simulink model "Function_Blocks"  (R2020b)
settings: Solver=FixedStepDiscrete  StartTime=0.0  StopTime=40  FixedStep=0.001  RelTol=1e-3
undefined symbols (not defined in the file): AA, C1, DiscIntNeverNeededParam, Error_Limit, kq, kqL
libraries: simulink x1, eeGeneralControl x1
(part 2 of 2)

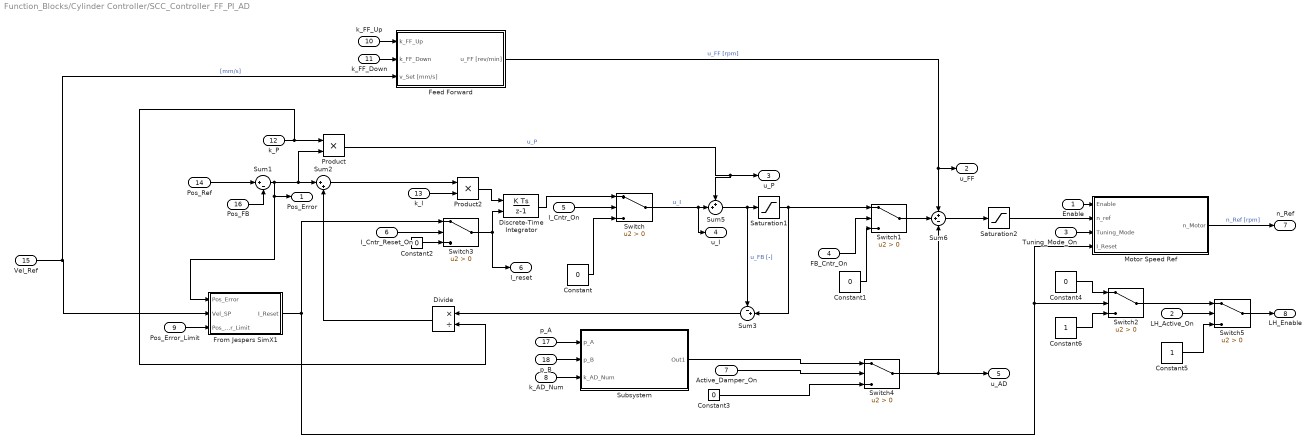
== system Function_Blocks/Cylinder Controller/SCC_Controller_FF_PI_AD ==
  Enable : Inport  OutDataTypeStr=boolean
  LH_Active_On : Inport  Port=2
  Tuning_Mode_On : Inport  Port=3  OutDataTypeStr=boolean
  FB_Cntr_On : Inport  Port=4  OutDataTypeStr=boolean
  I_Cntr_On : Inport  Port=5  OutDataTypeStr=boolean
  I_Cntr_Reset_On : Inport  Port=6  OutDataTypeStr=boolean
  Active_Damper_On : Inport  Port=7  OutDataTypeStr=boolean
  k_AD_Num : Inport  Port=8
  Pos_Error_Limit : Inport  Port=9
  k_FF_Up : Inport  Port=10
  k_FF_Down : Inport  Port=11
  k_P : Inport  Port=12
  k_I : Inport  Port=13
  Pos_Ref : Inport  Port=14
  Vel_Ref : Inport  Port=15
  Pos_FB : Inport  Port=16
  p_A : Inport  Port=17
  p_B : Inport  Port=18
  Constant{,1..3} (4 alike) : Constant  Value=0
  Constant4 : Constant  Value=0  OutDataTypeStr=boolean
  Constant5 : Constant  OutDataTypeStr=boolean
  Constant6 : Constant  OutDataTypeStr=boolean
  Discrete-Time Integrator : DiscreteIntegrator  ExternalReset=sampled level  SampleTime=0.001  ICPrevOutput=DiscIntNeverNeededParam  ICPrevScaledInput=DiscIntNeverNeededParam
  Divide : Product  Inputs=*/
  Feed Forward : Subsystem
  From Jespers SimX1 : MATLAB Function  TreatAsAtomicUnit=on
  Motor Speed Ref : MATLAB Function  TreatAsAtomicUnit=on
  Product : Product
  Product2 : Product
  Saturation1 : Saturate  UpperLimit=3500  LowerLimit=-3500
  Saturation2 : Saturate  UpperLimit=3500  LowerLimit=-3500
  Subsystem : Subsystem
  Sum1 : Sum  Inputs=|+-
  Sum2 : Sum  Inputs=|++
  Sum3 : Sum  Inputs=-+|
  Sum5 : Sum  Inputs=++|
  Sum6 : Sum  Inputs=++-
  Switch{,1..5} (6 alike) : Switch  Criteria=u2 > Threshold
  Pos_Error : Outport  VectorParamsAs1DForOutWhenUnconnected=off
  u_FF : Outport  Port=2  VectorParamsAs1DForOutWhenUnconnected=off
  u_P : Outport  Port=3  VectorParamsAs1DForOutWhenUnconnected=off
  u_I : Outport  Port=4  VectorParamsAs1DForOutWhenUnconnected=off
  u_AD : Outport  Port=5  VectorParamsAs1DForOutWhenUnconnected=off
  I_reset : Outport  Port=6  VectorParamsAs1DForOutWhenUnconnected=off
  n_Ref : Outport  Port=7  VectorParamsAs1DForOutWhenUnconnected=off
  LH_Enable : Outport  Port=8  OutDataTypeStr=boolean  VectorParamsAs1DForOutWhenUnconnected=off
  wires:
  Product2/1 -> Discrete-Time Integrator/1
  Pos_FB/1 -> Sum1/2
  Product/1 -> u_P/1, Sum5/1  "u_P"
  Sum2/1 -> Product2/1
  Divide/1 -> Sum2/2
  k_P/1 -> Divide/2, Product/1
  k_I/1 -> Product2/2
  Sum1/1 -> From Jespers SimX1/1(Pos_Error), Pos_Error/1, Product/2, Sum2/1
  Discrete-Time Integrator/1 -> Switch/1
  Switch/1 -> u_I/1, Sum5/2  "u_I"
  I_Cntr_On/1 -> Switch/2
  Constant/1 -> Switch/3
  Pos_Ref/1 -> Sum1/1
  Vel_Ref/1 -> Feed Forward/3(v_Set [mm/s]), From Jespers SimX1/2(Vel_SP)  "[mm/s]"
  Switch3/1 -> I_reset/1, Discrete-Time Integrator/2
  Saturation2/1 -> Motor Speed Ref/2(n_ref)
  Sum5/1 -> Sum3/1, Saturation1/1  "u_FB [-]"
  I_Cntr_Reset_On/1 -> Switch3/2
  Pos_Error_Limit/1 -> From Jespers SimX1/3(Pos_Error_Limit)
  Constant2/1 -> Switch3/3
  Constant3/1 -> Switch4/3
  Active_Damper_On/1 -> Switch4/2
  Switch4/1 -> Sum6/3, u_AD/1
  p_A/1 -> Subsystem/1(p_A)
  p_B/1 -> Subsystem/2(p_B)
  k_AD_Num/1 -> Subsystem/3(k_AD_Num)
  Subsystem/1(Out1) -> Switch4/1
  Tuning_Mode_On/1 -> Motor Speed Ref/3(Tuning_Mode)
  Motor Speed Ref/1(n_Motor) -> n_Ref/1  "n_Ref [rpm]"
  Sum3/1 -> Divide/1
  Sum6/1 -> Saturation2/1
  Feed Forward/1(u_FF [rev/min]) -> u_FF/1, Sum6/1  "u_FF [rpm]"
  Constant1/1 -> Switch1/3
  FB_Cntr_On/1 -> Switch1/2
  Saturation1/1 -> Switch1/1, Sum3/2
  Switch1/1 -> Sum6/2
  Constant5/1 -> Switch5/3
  LH_Active_On/1 -> Switch5/2
  Switch5/1 -> LH_Enable/1
  Enable/1 -> Motor Speed Ref/1(Enable)
  k_FF_Up/1 -> Feed Forward/1(k_FF_Up)
  k_FF_Down/1 -> Feed Forward/2(k_FF_Down)
  From Jespers SimX1/1(I_Reset) -> Switch2/2, Motor Speed Ref/4(I_Reset), Switch3/1
  Switch2/1 -> Switch5/1
  Constant4/1 -> Switch2/1
  Constant6/1 -> Switch2/3

== system Function_Blocks/Pressure_Feed_Forward/Subsystem2 ==
  p001 : Inport
  Trigger : TriggerPort  TriggerType=falling  VariantControl=Variant  PortDimensions=1
  p001_Hold : Outport  VectorParamsAs1DForOutWhenUnconnected=off
  wires:
  p001/1 -> p001_Hold/1

== system Function_Blocks/SCC_DPF/Subsystem ==
  pp : Inport
  pr : Inport  Port=2
  Trigger : TriggerPort  TriggerType=falling  VariantControl=Variant  PortDimensions=1
  pp0 : Outport  VectorParamsAs1DForOutWhenUnconnected=off
  pr0 : Outport  Port=2  VectorParamsAs1DForOutWhenUnconnected=off
  wires:
  pp/1 -> pp0/1
  pr/1 -> pr0/1

== system Function_Blocks/SCC_HPPF1/Subsystem2 ==
  pp : Inport
  pr : Inport  Port=2
  Trigger : TriggerPort  TriggerType=falling  VariantControl=Variant  PortDimensions=1
  pp0 : Outport  VectorParamsAs1DForOutWhenUnconnected=off
  pr0 : Outport  Port=2  VectorParamsAs1DForOutWhenUnconnected=off
  wires:
  pp/1 -> pp0/1
  pr/1 -> pr0/1

== system Function_Blocks/SCC_LPPF/Subsystem ==
  pp : Inport
  pr : Inport  Port=2
  Trigger : TriggerPort  TriggerType=falling  VariantControl=Variant  PortDimensions=1
  pp0 : Outport  VectorParamsAs1DForOutWhenUnconnected=off
  pr0 : Outport  Port=2  VectorParamsAs1DForOutWhenUnconnected=off
  wires:
  pp/1 -> pp0/1
  pr/1 -> pr0/1

== system Function_Blocks/Cylinder Controller/SCC_Controller_FF_PI_AD/Feed Forward ==
  k_FF_Up : Inport
  k_FF_Down : Inport  Port=2
  v_Set [mm/s] : Inport  Port=3
  Lift crane (pumping mode) : Product
  Lower crane (motoring mode) : Product
  Switch : Switch
  u_FF [rev/min] : Outport  VectorParamsAs1DForOutWhenUnconnected=off
  wires:
  Lower crane (motoring mode)/1 -> Switch/3  "[rev/min]"
  Lift crane (pumping mode)/1 -> Switch/1  "[rev/min]"
  Switch/1 -> u_FF [rev/min]/1
  v_Set [mm/s]/1 -> Lower crane (motoring mode)/1, Lift crane (pumping mode)/2, Switch/2
  k_FF_Up/1 -> Lift crane (pumping mode)/1
  k_FF_Down/1 -> Lower crane (motoring mode)/2

== system Function_Blocks/Cylinder Controller/SCC_Controller_FF_PI_AD/Subsystem ==
  p_A : Inport
  p_B : Inport  Port=2
  k_AD_Num : Inport  Port=3
  Cylinder Area Ratio : Gain  Gain=0.710059171597633
  Gain1 : Gain  Gain=-1
  Load Pressure : Sum  Inputs=|+-  OutDataTypeStr=double
  Scope : Scope
  Transfer Fcn1 1 : DiscreteTransferFcn  NumeratorSource=Input port  Numerator=[5e-5 -5e-05]  Denominator=[1 -0.997]  a0EqualsOne=on
      settings: InputPortMap=u0,p1
  Vector Concatenate : Concatenate
  Out1 : Outport  VectorParamsAs1DForOutWhenUnconnected=off
  wires:
  k_AD_Num/1 -> Vector Concatenate/1, Gain1/1
  Transfer Fcn1 1/1 -> Out1/1, Scope/1
  p_A/1 -> Load Pressure/1
  Vector Concatenate/1 -> Transfer Fcn1 1/2
  Cylinder Area Ratio/1 -> Load Pressure/2
  Load Pressure/1 -> Transfer Fcn1 1/1
  p_B/1 -> Cylinder Area Ratio/1
  Gain1/1 -> Vector Concatenate/2

== matlab function Function_Blocks/SCC_SinProfile/WaveSignal ==
  data: x0 input; v0 input; xC_SP input; Ts input; phi input; x output; t input; dx output
function [x,dx] = fcn(x0,v0,xC_SP,Ts,phi,t)

A=xC_SP/2;

x0=x0+A;
v0=v0;

x = x0+A*cos(2*pi*(1/Ts)*t+phi);
dx = v0-2*pi*A*(1/Ts)*sin(2*pi*(1/Ts)*t+phi);

== matlab function Function_Blocks/SCC_Cascaded_Controller/Controller_Reset ==
  data: Clock input; I_Reset output
function I_Reset = fcn(Clock)

I_Reset = 1;

if Clock > 0
   I_Reset = 0;
else
    I_Reset = 1;
end

== matlab function Function_Blocks/LHV_Enabler/MATLAB Function1 ==
  data: y output; LHC_error input; LHC_error_SP input; SM_ON input
function y = fcn(LHC_error, LHC_error_SP, SM_ON)


if SM_ON > 0 && abs(LHC_error)  < LHC_error_SP
y = 1;  
else 
y = 0;
end

== matlab function Function_Blocks/Pressure_Feed_Forward/MATLAB Function1 ==
  data: FeedBackPressureTerm output; p001_Hold input; p_32 input; x_dot_ref input
function FeedBackPressureTerm = fcn(p001_Hold,p_32,x_dot_ref)

if (p001_Hold - p_32) <= 0
FeedBackPressureTerm = 0;
elseif abs(x_dot_ref) > 0.0003
FeedBackPressureTerm = 0;
else
FeedBackPressureTerm =  6.0256*10^(-5)/2 * (p001_Hold - p_32);
end

== matlab function Function_Blocks/VCC_Pos_Step/StepFunction ==
  data: x0 input; x_SP input; t0 input; t1 input; t input; y output
function y  = step(x0,x_SP, t0,t1,  t)


if t>=0 && t<t0
    y = x0;
elseif t>=(t0) && t<(t0+t1)
    y = x_SP;
else
    y = x0; 
end

== matlab function Function_Blocks/S_shape_Profile/SP_Generator ==
  data: PositionRef output; VelocityRef output; AccelerationRef output; JerkRef output; InPositionTime output; s0 input; v0 input; Desired_Position input; VelocitySP input; t0 input; HoldPositionTime input; t input; Error output
function [PositionRef,VelocityRef,AccelerationRef,JerkRef, InPositionTime, Error] = fcn(s0,v0, Desired_Position,VelocitySP, t0,HoldPositionTime,t)


PositionSP = Desired_Position - s0;

a0 = 0;
j0 = 0;
AccelerationSP = VelocitySP;

vel=VelocitySP;
as=AccelerationSP;
% Input velocity 
vs=vel; %[rad/s]
% Delta velocity 
dv=(vs-v0); %[rad/s]     
% Max Jerk Considerations
jm=as^2/dv; %%[rad/s^3] 
% Constant Velocity periodes
s_acc=(vs^2-v0^2)/as;
CstVelTime=(PositionSP-2*s_acc)/vs;
if CstVelTime < 0
Error = 1;
else 
Error = 0;
end

% Time periodes,
t1=t0+(as/jm);
t2=t1+(as/jm);
t3=t2+CstVelTime;
t4=t3+(as/jm);
t5=t4+(as/jm);
t6=t5+HoldPositionTime;
t7=t6+(as/jm);
t8=t7+(as/jm);
t9=t8+CstVelTime;
t10=t9+(as/jm);
t11=t10+(as/jm);
% Position and Velocity Constants
sh=(v0+(as^2)/(6*jm))*(as/jm);
vh=(vs-v0)/2;
s3=s_acc+vs*(t3-t2);
s4=s3+vs*(t4-t3)-jm*((t4-t3)^3)/6;
v4=vs-jm*((t4-t3)^2)/2;
s5=s0+jm*((t5-t4)^3)/6-as*((t5-t4)^2)/2+v4*(t5-t4)+s4;
%s6=s5+(s0+v0*(t7-t6)+jm*((t7-t6)^3)/6);
s7= s5-(s_acc+vs*(t9-t8));
s8= s7-(vs*(t10-t9)-jm*((t10-t9)^3)/6);
%s9= s8-(jm*((t11-t10)^3)/6-as*((t11-t10)^2)/2+v4*(t11-t10));
%Phase0
if  Error == 1   
s = s0;
v = v0;
a = a0;
j=j0; 
elseif  (t >= 0) && (t <= t0)    
s = s0;
v = v0;
a = a0;
j=j0;        
%Phase1 - concave Acc
elseif  (t >= t0) && (t <= (t1))
s = s0+v0*(t-t0)+jm*((t-t0)^3)/6;
v = v0+jm*((t-t0)^2)/2;
a = jm*(t-t0);
j=jm;
%Phase2 - convex Acc
elseif (t >= (t1)) && (t <= (t2))
s = s0+sh+vh*(t-t1)+as*((t-t1)^2)/2-jm*((t-t1)^3)/6;
v = vh+as*(t-t1)-jm*((t-t1)^2)/2;
a = as-jm*(t-t1);
j = -jm; 
%Phase3 - constant velocity
elseif (t >= t2) && (t <= t3)
s = s0+s_acc+vs*(t-t2);
v = vs;
a = 0;
j = 0;   
%Phase4 - convex Dec
elseif (t >= t3) && (t <= t4)
s = s0+s3+vs*(t-t3)-jm*((t-t3)^3)/6;
v = vs-jm*((t-t3)^2)/2;
a = -jm*(t-t3);
j = -jm; 
%Phase5 - concav Dec
elseif (t >= t4) && (t <= t5)
s = s0+jm*((t-t4)^3)/6-as*((t-t4)^2)/2+v4*(t-t4)+s4;
v = jm*((t-t4)^2)/2-as*(t-t4)+v4;
a = jm*(t-t4)-as;
j=jm; 
%Phase6 - holding position
elseif (t >= t5) && (t <= t6)
s = s5;
v = 0;
a = 0;
j = 0;  
%Phase7 - concave Dec
elseif (t >= t6) && (t <= t7)
s = s5-(v0*(t-t6)+jm*((t-t6)^3)/6);
v = -(v0+jm*((t-t6)^2)/2);
a = -jm*(t-t6);
j=-jm;
%Phase8 - convex Dec
elseif (t >= t7) && (t <= t8)    
s = s5-(sh+vh*(t-t7)+as*((t-t7)^2)/2-jm*((t-t7)^3)/6);
v = -(vh+as*(t-t7)-jm*((t-t7)^2)/2);
a = -(as-jm*(t-t7));
j = jm; 
%Phase9 - constant velocity
elseif (t >= t8) && (t <= t9)
s = s5-(s_acc+vs*(t-t8));
v = -vs;
a = 0;
j = 0;     
%Phase10 - concav Acc
elseif (t >= t9) && (t <= t10)
s = s7-(vs*(t-t9)-jm*((t-t9)^3)/6);
v = -(vs-jm*((t-t9)^2)/2);
a = jm*(t-t9);
j = jm; 
%Phase11 - convex Acc
elseif (t >= t10) && (t <= t11)
s = s8-(jm*((t-t10)^3)/6-as*((t-t10)^2)/2+v4*(t-t10));
v = -(jm*((t-t10)^2)/2-as*(t-t10)+v4);
a = -(jm*(t-t10)-as);
j=-jm; 
%Phase12 - hold position
else
s = s0;
v = v0;
a = a0;
j = j0;
end

if t == 0
PositionRef=s0; %[mm]
else 
PositionRef=s; %[mm]
end 

InPositionTime=t5; %[s]
VelocityRef=v; %[mm/s]
AccelerationRef=a; %[mm/s^2]
JerkRef=j; % %[mm/s^3]

== matlab function Function_Blocks/Ramp_Profile/WaveSignal ==
  data: x0 input; v0 input; x_ref input; x output; v_ref input; t0 input; tRamp input; tWait input; v output; t input; T output; Error output
function [x,v,T, Error] = fcn(x0,v0, x_ref,v_ref,t0,tRamp,tWait,t)
x_SP = x_ref - x0;
vs=v_ref;
slopeExt=v0-vs;
slopeRetr=-vs-v0;

as = vs/tRamp;
s_acc=(vs^2-v0^2)/as;

tHold=(x_SP-s_acc)/vs;

if tHold < 0 
Error = 1;
else 
Error = 0;
end

t1=tRamp;
t2=tHold; 
t3=tRamp;
t4=tWait;
t5=t1;
t6=t2;
t7=t3;

x = x0;
x1 = x0 + v0*((t0+t1)-t0)-(slopeExt/t1)*((t0+t1)-t0)^2/2;
x2 = x1 + vs*((t0+t1+t2)-(t0+t1)); 
x4 = x_ref - v0*((t0+t1+t2+t3+t4+t5)-(t0+t1+t2+t3+t4))+(slopeRetr/t5)*((t0+t1+t2+t3+t4+t5)-(t0+t1+t2+t3+t4))^2/2; 
x5 = x4-vs*((t0+t1+t2+t3+t4+t5+t6)-(t0+t1+t2+t3+t4+t5));  

if Error == 1
x = x0;
v = v0; 
elseif t>=0 && t<t0
x = x0; 
v = v0;
elseif t>=t0 && t<(t0+t1)
x = x0 + v0*(t-t0)-(slopeExt/t1)*(t-t0)^2/2;
v = v0-(slopeExt/t1)*(t-t0);  
elseif t>=(t0+t1) && t<(t0+t1+t2)
x = x1 + vs*(t-(t0+t1)); 
v = vs; 
elseif t>=(t0+t1+t2) && t<(t0+t1+t2+t3)
x = x2+vs*(t-(t0+t1+t2))+(slopeExt/t3)*(t-(t0+t1+t2))^2/2; 
v = vs+(slopeExt/t3)*(t-(t0+t1+t2));   
elseif t>=(t0+t1+t2+t3) && t<(t0+t1+t2+t3+t4)
x = x_ref;
v = v0;  
elseif t>=(t0+t1+t2+t3+t4) && t<(t0+t1+t2+t3+t4+t5)
x = x_ref - v0*(t-(t0+t1+t2+t3+t4))+(slopeRetr/t5)*(t-(t0+t1+t2+t3+t4))^2/2; 
v = v0+(slopeRetr/t5)*(t-(t0+t1+t2+t3+t4));     
elseif t>=(t0+t1+t2+t3+t4+t5) && t<(t0+t1+t2+t3+t4+t5+t6)
x = x4-vs*(t-(t0+t1+t2+t3+t4+t5));   
v = -vs;    
elseif t>=(t0+t1+t2+t3+t4+t5+t6) && t<(t0+t1+t2+t3+t4+t5+t6+t7)
x = x5-vs*(t-(t0+t1+t2+t3+t4+t5+t6))-(slopeRetr/t3)*(t-(t0+t1+t2+t3+t4+t5+t6))^2/2;    
v = -vs-(slopeRetr/t3)*(t-(t0+t1+t2+t3+t4+t5+t6));     
else 
x = x0;
v = v0; 
end

T = t0+t1+t2+t3+t4+t5+t6+t7;

== matlab function Function_Blocks/Cylinder Controller/SCC_Controller_FF_PI_AD/Motor Speed Ref ==
  data: Enable input; n_ref input; Tuning_Mode input; n_Motor output; I_Reset input
function n_Motor = fcn(Enable, n_ref, Tuning_Mode, I_Reset)


n_Motor = 0;

if Enable == 0
    n_Motor = 0; 
elseif (I_Reset == 0) 
    n_Motor = n_ref;  
elseif (Tuning_Mode == 1) 
    n_Motor = n_ref; 
else
   n_Motor = 0;
end

== matlab function Function_Blocks/Cylinder Controller/SCC_Controller_FF_PI_AD/From Jespers SimX1 ==
  data: Pos_Error input; Vel_SP input; Pos_Error_Limit input; I_Reset output
function I_Reset = fcn(Pos_Error, Vel_SP, Pos_Error_Limit)

I_Reset = 1;

if (abs(Pos_Error) <= Pos_Error_Limit) && (Vel_SP == 0)
   I_Reset = 1;
else
    I_Reset = 0;
end

== matlab function Function_Blocks/Motion_Reference_Generator_S_shape_Profile/SP_Generator ==
  data: PositionRef output; VelocityRef output; InPositionTime output; s0 input; v0 input; Desired_Position input; VelocitySP input; t0 input; HoldPositionTime input; t input; Error output
function [PositionRef,VelocityRef, InPositionTime, Error] = fcn(s0,v0, Desired_Position,VelocitySP, t0,HoldPositionTime,t)


PositionSP = Desired_Position - s0;

a0 = 0;
j0 = 0;
AccelerationSP = VelocitySP;

vel=VelocitySP;
as=AccelerationSP;
% Input velocity 
vs=vel; %[rad/s]
% Delta velocity 
dv=(vs-v0); %[rad/s]     
% Max Jerk Considerations
jm=as^2/dv; %%[rad/s^3] 
% Constant Velocity periodes
s_acc=(vs^2-v0^2)/as;
CstVelTime=(PositionSP-2*s_acc)/vs;
if CstVelTime < 0
Error = 1;
else 
Error = 0;
end

% Time periodes,
t1=t0+(as/jm);
t2=t1+(as/jm);
t3=t2+CstVelTime;
t4=t3+(as/jm);
t5=t4+(as/jm);
t6=t5+HoldPositionTime;
t7=t6+(as/jm);
t8=t7+(as/jm);
t9=t8+CstVelTime;
t10=t9+(as/jm);
t11=t10+(as/jm);
% Position and Velocity Constants
sh=(v0+(as^2)/(6*jm))*(as/jm);
vh=(vs-v0)/2;
s3=s_acc+vs*(t3-t2);
s4=s3+vs*(t4-t3)-jm*((t4-t3)^3)/6;
v4=vs-jm*((t4-t3)^2)/2;
s5=s0+jm*((t5-t4)^3)/6-as*((t5-t4)^2)/2+v4*(t5-t4)+s4;
%s6=s5+(s0+v0*(t7-t6)+jm*((t7-t6)^3)/6);
s7= s5-(s_acc+vs*(t9-t8));
s8= s7-(vs*(t10-t9)-jm*((t10-t9)^3)/6);
%s9= s8-(jm*((t11-t10)^3)/6-as*((t11-t10)^2)/2+v4*(t11-t10));
%Phase0
if  Error == 1   
s = s0;
v = v0;
a = a0;
j=j0; 
elseif  (t >= 0) && (t <= t0)    
s = s0;
v = v0;
a = a0;
j=j0;        
%Phase1 - concave Acc
elseif  (t >= t0) && (t <= (t1))
s = s0+v0*(t-t0)+jm*((t-t0)^3)/6;
v = v0+jm*((t-t0)^2)/2;
a = jm*(t-t0);
j=jm;
%Phase2 - convex Acc
elseif (t >= (t1)) && (t <= (t2))
s = s0+sh+vh*(t-t1)+as*((t-t1)^2)/2-jm*((t-t1)^3)/6;
v = vh+as*(t-t1)-jm*((t-t1)^2)/2;
a = as-jm*(t-t1);
j = -jm; 
%Phase3 - constant velocity
elseif (t >= t2) && (t <= t3)
s = s0+s_acc+vs*(t-t2);
v = vs;
a = 0;
j = 0;   
%Phase4 - convex Dec
elseif (t >= t3) && (t <= t4)
s = s0+s3+vs*(t-t3)-jm*((t-t3)^3)/6;
v = vs-jm*((t-t3)^2)/2;
a = -jm*(t-t3);
j = -jm; 
%Phase5 - concav Dec
elseif (t >= t4) && (t <= t5)
s = s0+jm*((t-t4)^3)/6-as*((t-t4)^2)/2+v4*(t-t4)+s4;
v = jm*((t-t4)^2)/2-as*(t-t4)+v4;
a = jm*(t-t4)-as;
j=jm; 
%Phase6 - holding position
elseif (t >= t5) && (t <= t6)
s = s5;
v = 0;
a = 0;
j = 0;  
%Phase7 - concave Dec
elseif (t >= t6) && (t <= t7)
s = s5-(v0*(t-t6)+jm*((t-t6)^3)/6);
v = -(v0+jm*((t-t6)^2)/2);
a = -jm*(t-t6);
j=-jm;
%Phase8 - convex Dec
elseif (t >= t7) && (t <= t8)    
s = s5-(sh+vh*(t-t7)+as*((t-t7)^2)/2-jm*((t-t7)^3)/6);
v = -(vh+as*(t-t7)-jm*((t-t7)^2)/2);
a = -(as-jm*(t-t7));
j = jm; 
%Phase9 - constant velocity
elseif (t >= t8) && (t <= t9)
s = s5-(s_acc+vs*(t-t8));
v = -vs;
a = 0;
j = 0;     
%Phase10 - concav Acc
elseif (t >= t9) && (t <= t10)
s = s7-(vs*(t-t9)-jm*((t-t9)^3)/6);
v = -(vs-jm*((t-t9)^2)/2);
a = jm*(t-t9);
j = jm; 
%Phase11 - convex Acc
elseif (t >= t10) && (t <= t11)
s = s8-(jm*((t-t10)^3)/6-as*((t-t10)^2)/2+v4*(t-t10));
v = -(jm*((t-t10)^2)/2-as*(t-t10)+v4);
a = -(jm*(t-t10)-as);
j=-jm; 
%Phase12 - hold position
else
s = s0;
v = v0;
a = a0;
j = j0;
end

if t == 0
PositionRef=s0; %[mm]
else 
PositionRef=s; %[mm]
end 

InPositionTime=t5; %[s]
VelocityRef=v; %[mm/s]
AccelerationRef=a; %[mm/s^2]
JerkRef=j; % %[mm/s^3]

== matlab function Function_Blocks/SCC_PFB_Controller_PID/Controller_Reset ==
  data: Clock input; I_Reset output
function I_Reset = fcn(Clock)

I_Reset = 1;

if Clock > 0
   I_Reset = 0;
else
    I_Reset = 1;
end

== matlab function Function_Blocks/SCC_Controller_PFB/Controller_Reset ==
  data: Clock input; I_Reset output
function I_Reset = fcn(Clock)

I_Reset = 1;

if Clock > 0
   I_Reset = 0;
else
    I_Reset = 1;
end

== matlab function Function_Blocks/SCC_PFB_Controller_PID2/Controller_Reset ==
  data: Clock input; I_Reset output
function I_Reset = fcn(Clock)

I_Reset = 1;

if Clock > 0
   I_Reset = 0;
else
    I_Reset = 1;
end
